simulink model "readingP300_corr"  (R2021b)
settings: Solver=FixedStepAuto  StartTime=0.0  StopTime=10  FixedStep=0.004  RelTol=1e-3
undefined symbols (not defined in the file or in its folder): UN
libraries: UnicornLib x1
settings Model: Creator=s206180  LastModifiedBy=s206180
settings SolverCC: AlgebraicLoopSolver=TrustRegion
settings DataIOCC: ReturnWorkspaceOutputs=off
settings DebuggingCC: SFMachineParentedDataDiag=warning  ArithmeticOperatorsInVariantConditions=warning
settings SFSimCC: SimUseLocalCustomCode=off  CustomCodeUndefinedFunction=UseInterfaceOnly
settings RTWCC: RTWUseLocalCustomCode=off
settings CodeAppCC: StateflowObjectComments=on

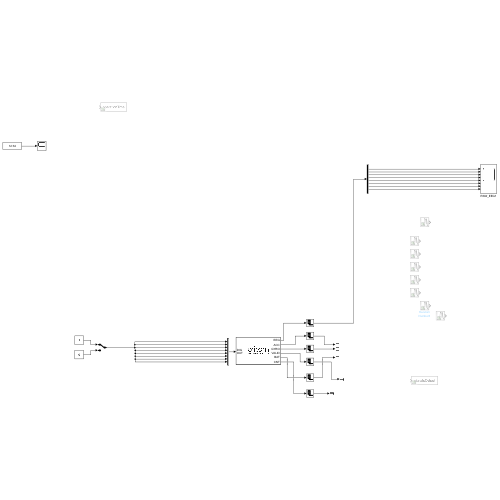
[thumbnail: Simulink's stored preview of the top-level diagram]
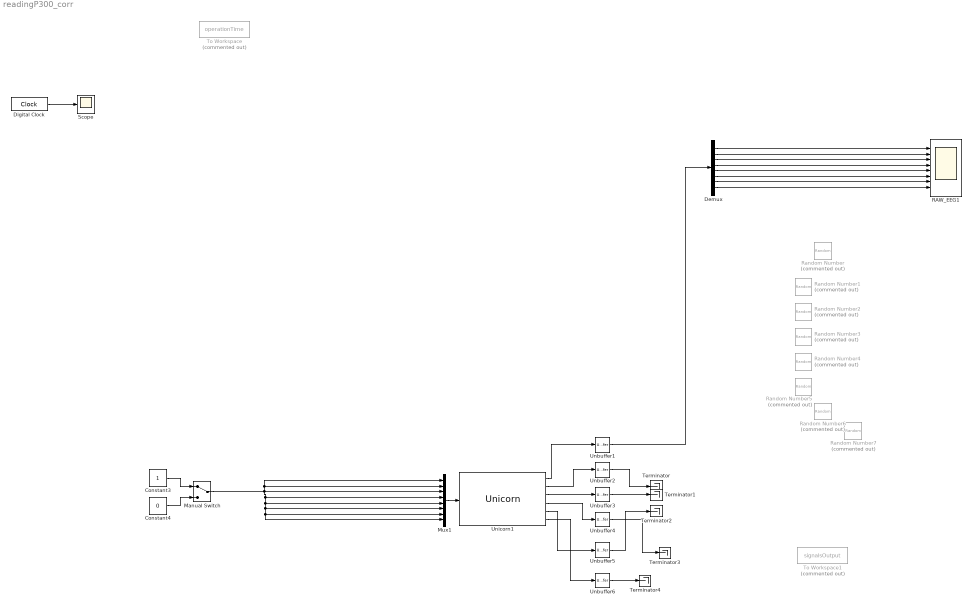
== system readingP300_corr ==
  Constant3 : Constant  OutDataTypeStr=boolean
  Constant4 : Constant  Value=0  OutDataTypeStr=boolean
  Demux : Demux  Outputs=8
  Digital Clock : DigitalClock  SampleTime=0.1
  Manual Switch : ManualSwitch
  Mux1 : Mux  Inputs=8
  RAW_EEG1 : Scope  NumInputPorts=8
  Random Number{,1..7} (8 alike) : RandomNumber  Commented=on  SampleTime=0.004
  Scope : Scope
  Terminator{,1..4} (5 alike) : Terminator
  To Workspace : ToWorkspace  Commented=on  VariableName=operationTime  SaveFormat=Structure  SampleTime=-1
  To Workspace1 : ToWorkspace  Commented=on  VariableName=signalsOutput  SaveFormat=Structure With Time  SampleTime=-1
  Unbuffer{1..6} (6 alike) : Unbuffer
  Unicorn1 : UnicornLib/Unicorn  serial=UN-2019.08.19  old_serial=UN-2019.08.19  frame_length=1  input_source=Electrode
      settings: SourceProductName=Unicorn
  wires:
  Constant3/1 -> Manual Switch/1
  Mux1/1 -> Unicorn1/1
  Unbuffer2/1 -> Terminator/1
  Constant4/1 -> Manual Switch/2
  Manual Switch/1 -> Mux1/4, Mux1/5, Mux1/6, Mux1/7, Mux1/8, Mux1/3, Mux1/2, Mux1/1
  Unbuffer3/1 -> Terminator1/1
  Unbuffer5/1 -> Terminator2/1
  Unbuffer4/1 -> Terminator3/1
  Unbuffer6/1 -> Terminator4/1
  Digital Clock/1 -> Scope/1
  Unicorn1/1 -> Unbuffer1/1
  Unicorn1/2 -> Unbuffer2/1
  Unicorn1/3 -> Unbuffer3/1
  Unicorn1/4 -> Unbuffer4/1
  Unicorn1/5 -> Unbuffer5/1
  Unicorn1/6 -> Unbuffer6/1
  Unbuffer1/1 -> Demux/1
  Demux/1 -> RAW_EEG1/1
  Demux/2 -> RAW_EEG1/2
  Demux/3 -> RAW_EEG1/3
  Demux/4 -> RAW_EEG1/4
  Demux/5 -> RAW_EEG1/5
  Demux/6 -> RAW_EEG1/6
  Demux/7 -> RAW_EEG1/7
  Demux/8 -> RAW_EEG1/8
